simulink model "CrazyFlie_PosCntrl"  (R2015a)
settings: Solver=FixedStepDiscrete  SolverMode=SingleTasking  StartTime=0.0  StopTime=inf  FixedStep=0.02  RelTol=1e-3
PreLoadFcn:
  | addpath([cd filesep 'QuadCom']);
InitFcn:
  | %cd('..\Uart_Com');
libraries: simulink x2, CrazyFlie_lib x2
settings Model: CovSFcnEnable=off  Creator=Michael  LastModifiedBy=rshum
settings DataIOCC: SignalLoggingSaveFormat=ModelDataLogs
settings OptimizationCC: ExpressionDepthLimit=2147483647
settings DebuggingCC: UnderspecifiedInitializationDetection=Classic  MergeDetectMultiDrivingBlocksExec=none  SolverPrmCheckMsg=warning  FcnCallInpInsideContextMsg=UseLocalSettings  StateNameClashWarn=warning
settings HardwareCC: ProdLargestAtomicInteger=Long  ProdLargestAtomicFloat=Float  ProdHWDeviceType=ARM Compatible->ARM 7
settings SFSimCC: SimParseCustomCode=off
settings GRTTargetCC: CombineOutputUpdateFcns=off  GRTInterface=on

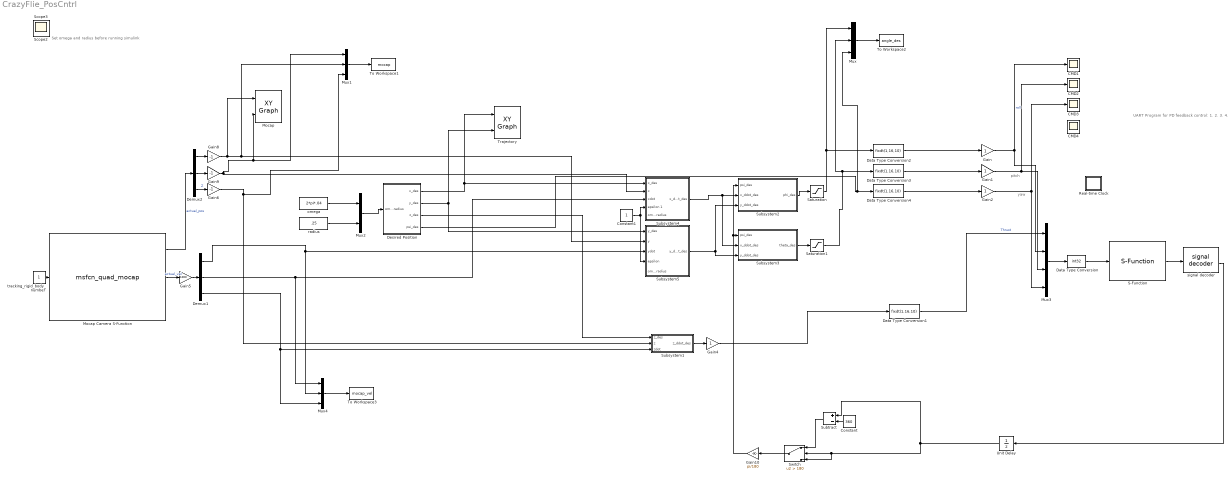
== system CrazyFlie_PosCntrl ==
  note: yaw
  note: pitch
  note: Set omega and radius before running simulink
  note: UART Program for PD feedback control:
      | 1.
      | 2.
      | 3.
      | 4.
  CMD{1..4} (4 alike) : Scope
      CMD1 settings: YMin=-1  YMax=1  SaveName=ScopeData15
      CMD2 settings: YMin=-0.15  YMax=0.15  SaveName=ScopeData16
      CMD3 settings: YMin=11.875  YMax=11.875  SaveName=ScopeData17
      CMD4 settings: YMin=11.875  YMax=11.875  SaveName=ScopeData18
  Constant : Constant  Value=360
  Constant1 : Constant
  Data Type Conversion : DataTypeConversion  OutDataTypeStr=int32  ConvertRealWorld=Stored Integer (SI)  SaturateOnIntegerOverflow=on
  Data Type Conversion{1..4} (4 alike) : DataTypeConversion  OutDataTypeStr=fixdt(1,16,10)
  Demux1 : Demux  Outputs=3
  Demux2 : Demux  Outputs=3
  "Desired Position " : Subsystem
  Gain : Gain  OutDataTypeStr=fixdt(1,16,10)
  Gain1 : Gain  OutDataTypeStr=fixdt(1,16,10)
  Gain10 : Gain  Gain=pi/180
  Gain2 : Gain  OutDataTypeStr=fixdt(1,16,10)
  Gain4 : Gain
  Gain5 : Gain  Gain=1000
  Gain6 : Gain  Gain=-1
  Gain8 : Gain  Gain=-1
  Gain9 : Gain  Gain=-1
  Mocap : simulink/Sinks/XY Graph  xmin=-1  xmax=1  ymin=-1  ymax=1  st=-1
  Mocap Camera S-Function : M-S-Function  FunctionName=msfcn_quad_mocap  mask(Mocap-Motion-Track){}
      mask Display:
      | image(imread('camera.png'))
      | color('white')
      | port_label('output', 1, 'Quad_Pos')
      | port_label('output', 2, 'Quad_Vel')
      | port_label('output', 3, 'Rel_Yaw')
      | port_label('input', 1, 'trackingBody_Num')
  Mux : Mux  Inputs=3
  Mux1 : Mux  Inputs=3
  Mux2 : Mux  Inputs=2
  Mux3 : Mux
  Mux4 : Mux  Inputs=3
  Real-time Clock : Subsystem  mask(Real-time Clock){sample_time=0.02, tolerance=1}
      mask prompts: sample_time "Synchronize with real-time every n seconds:"; tolerance "Real-time warning tolerance (seconds):"
      mask help: Real-time Synchronization Block
      mask Help: This block synchronizes simulation time with the PC real-time clock or UNIX system clock. The first dialog entry is the period at which the clock is checked to insure real-time synchronization. The second dialog entry is the number of seconds that the simulation time must be within real-time before a warning is printed.
      mask Display: plot(0,0,100,100,[40,60,60,54,54,64,69,76,82,77,81,83,83,81,78,74,70,64,57,49,41,35,32,30,30,31,34,40,47,47,40,40],[90,90,85,85,80,79,76,87,80,70,64,57,49,41,33,28,24,22,21,23,25,31,37,46,56,65,73,78,80,85,85,90],[69,53,53],[64,50,73])
  S-Function : CrazyFlie_lib/S-Function
  Saturation : Saturate  UpperLimit=1  LowerLimit=-1
  Saturation1 : Saturate  UpperLimit=1  LowerLimit=-1
  Subsystem1 : Subsystem
  Subsystem2 : Subsystem
  Subsystem3 : Subsystem
  Subsystem4 : Subsystem
  Subsystem5 : Subsystem
  Subtract : Sum  Inputs=+-
  Switch : Switch  Criteria=u2 > Threshold  Threshold=180
  To Workspace1 : ToWorkspace  VariableName=mocap  SaveFormat=Timeseries  SampleTime=-1
  To Workspace2 : ToWorkspace  VariableName=angle_des  SaveFormat=Timeseries  SampleTime=-1
  To Workspace3 : ToWorkspace  VariableName=mocap_vel  SaveFormat=Timeseries  SampleTime=-1
  "Trajectory " : simulink/Sinks/XY Graph  xmin=-1  xmax=1  ymin=-1  ymax=1  st=-1
  Unit Delay : UnitDelay  SampleTime=-1
  omega : Constant  Value=2*pi*.04
  radius : Constant  Value=.25
  signal decoder : CrazyFlie_lib/signal decoder
  tracking_rigid_body_number : Constant
  Scope2 : Scope
      settings: YMin=-0.09  YMax=0.07  SaveName=ScopeData2  MaxDataPoints=7500
  Scope3 : Scope
      settings: YMin=-1.25  YMax=2.75  SaveName=ScopeData3  MaxDataPoints=7500
  wires:
  Data Type Conversion/1 -> S-Function/1
  Mux3/1 -> Data Type Conversion/1
  Data Type Conversion2/1 -> Gain/1
  Data Type Conversion3/1 -> Gain1/1
  Data Type Conversion4/1 -> Gain2/1
  Gain/1 -> Mux3/2, CMD1/1  "roll"
  Gain1/1 -> Mux3/3, CMD2/1
  Gain2/1 -> Mux3/4, CMD3/1
  "Desired Position "/3(z_des) -> Subsystem1/1(z_des)
  Demux2/3 -> Gain6/1  "Z"
  Subsystem4/1(x_ddot_des) -> Subsystem3/2(x_ddot_des), Subsystem2/2(x_ddot_des)
  Subsystem5/1(y_ddot_des) -> Subsystem2/3("y_ddot_des "), Subsystem3/3("y_ddot_des ")
  "Desired Position "/2(y_des) -> "Trajectory "/2, Subsystem5/1(y_des)
  "Desired Position "/1(x_des) -> "Trajectory "/1, Subsystem4/1(x_des)
  Demux2/1 -> Gain8/1
  Demux2/2 -> Gain9/1
  tracking_rigid_body_number/1 -> Mocap Camera S-Function/1
  Mocap Camera S-Function/1 -> Demux2/1  "actual_pos"
  Mocap Camera S-Function/2 -> Gain5/1  "actual_vel"
  Subsystem3/1("theta_des ") -> Saturation1/1
  Subsystem2/1("phi_des ") -> Saturation/1
  Gain8/1 -> Mocap/1, Mux1/2, Subsystem5/2(y)
  Gain9/1 -> Mocap/2, Mux1/1, Subsystem4/2(x)
  Mux1/1 -> To Workspace1/1
  Demux1/1 -> Mux4/2, Subsystem5/3("ydot ")
  Demux1/2 -> Mux4/1, Subsystem4/3("xdot ")
  Gain5/1 -> Demux1/1
  Gain6/1 -> Subsystem1/2(z), Mux1/3
  Subsystem1/1(z_ddot_des) -> Gain4/1
  Mux4/1 -> To Workspace3/1
  signal decoder/3 -> Unit Delay/1
  Constant/1 -> Subtract/2
  Subtract/1 -> Switch/1
  Switch/1 -> Gain10/1
  Gain10/1 -> Subsystem3/1("psi_des "), Subsystem2/1("psi_des ")
  Unit Delay/1 -> Switch/3, Switch/2, Subtract/1
  Constant1/1 -> Subsystem4/4(epsilon 1), Subsystem5/4("epsilon ")
  Mux/1 -> To Workspace2/1
  "Desired Position "/4(psi_des) -> Mux/3, Data Type Conversion4/1
  Saturation1/1 -> Data Type Conversion3/1, Mux/2
  Saturation/1 -> Data Type Conversion2/1, Mux/1
  Demux1/3 -> Mux4/3, Subsystem1/3("zdot ")
  Data Type Conversion1/1 -> Mux3/1  "Thrust"
  Gain4/1 -> Data Type Conversion1/1
  Mux2/1 -> "Desired Position "/1("omg_radius ")
  omega/1 -> Mux2/1
  radius/1 -> Mux2/2
  S-Function/1 -> signal decoder/1

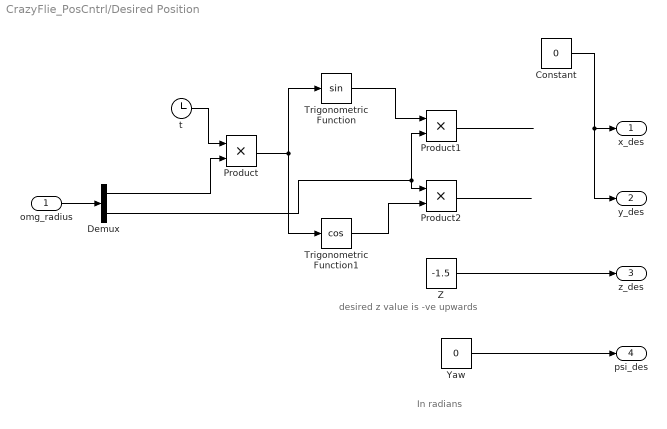
== system CrazyFlie_PosCntrl/Desired Position  ==
  note: desired z value
      | is -ve upwards
  note: In radians
  "omg_radius " : Inport
  Constant : Constant  Value=0
  Demux : Demux  Outputs=2
  Product : Product
  Product1 : Product
  Product2 : Product
  Trigonometric Function : Trigonometry
  Trigonometric Function1 : Trigonometry  Operator=cos
  Yaw : Constant  Value=0
  "Z " : Constant  Value=-1.5
  t : Clock
  x_des : Outport
  y_des : Outport  Port=2
  z_des : Outport  Port=3
  psi_des : Outport  Port=4
  wires:
  Yaw/1 -> psi_des/1
  "Z "/1 -> z_des/1
  Product2/1 -> ?
  Product1/1 -> ?
  t/1 -> Product/1
  Demux/1 -> Product/2
  Product/1 -> Trigonometric Function1/1, Trigonometric Function/1
  Demux/2 -> Product1/2, Product2/1
  Trigonometric Function/1 -> Product1/1
  Trigonometric Function1/1 -> Product2/2
  "omg_radius "/1 -> Demux/1
  Constant/1 -> y_des/1, x_des/1

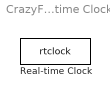
== system CrazyFlie_PosCntrl/Real-time Clock ==
  Real-time Clock : S-Function  FunctionName=rtclock  Parameters=sample_time, tolerance

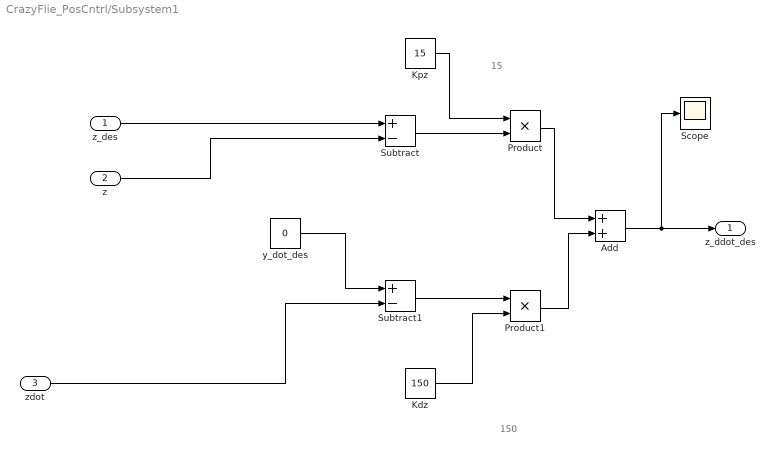
== system CrazyFlie_PosCntrl/Subsystem1 ==
  note: 15
  note: 150
  z_des : Inport
  z : Inport  Port=2
  "zdot " : Inport  Port=3
  Add : Sum
  "Kdz " : Constant  Value=150
  "Kpz " : Constant  Value=15
  Product : Product
  Product1 : Product
  Scope : Scope
      settings: YMin=-3  YMax=3  SaveName=ScopeData31
  Subtract : Sum  Inputs=+-
  Subtract1 : Sum  Inputs=+-
  y_dot_des : Constant  Value=0
  z_ddot_des : Outport
  wires:
  z/1 -> Subtract/2
  z_des/1 -> Subtract/1
  "Kpz "/1 -> Product/1
  Subtract/1 -> Product/2
  y_dot_des/1 -> Subtract1/1
  Subtract1/1 -> Product1/1
  "Kdz "/1 -> Product1/2
  Product1/1 -> Add/2
  Product/1 -> Add/1
  Add/1 -> Scope/1, z_ddot_des/1
  "zdot "/1 -> Subtract1/2

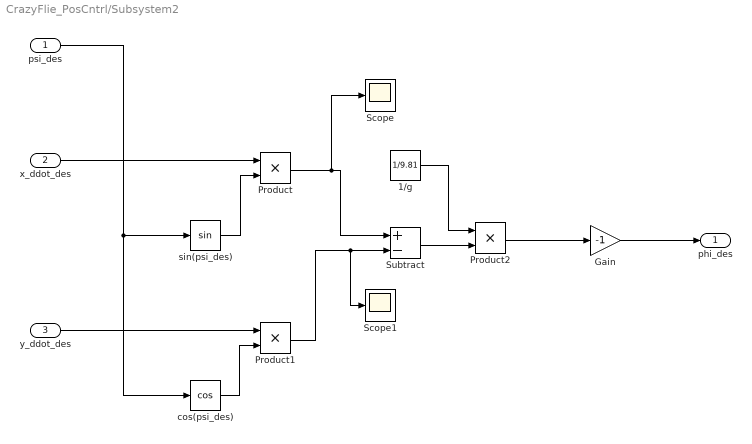
== system CrazyFlie_PosCntrl/Subsystem2 ==
  "psi_des " : Inport
  x_ddot_des : Inport  Port=2
  "y_ddot_des " : Inport  Port=3
  "1/g " : Constant  Value=1/9.81
  Gain : Gain  Gain=-1
  Product : Product
  Product1 : Product
  Product2 : Product
  Scope : Scope
      settings: TimeRange=30  YMin=-30  YMax=20  SaveName=ScopeData28
  Scope1 : Scope
      settings: TimeRange=30  YMin=-61.5  YMax=-61.3  SaveName=ScopeData30
  Subtract : Sum  Inputs=+-
  cos(psi_des) : Trigonometry  Operator=cos
  sin(psi_des) : Trigonometry
  "phi_des " : Outport
  wires:
  "psi_des "/1 -> sin(psi_des)/1, cos(psi_des)/1
  x_ddot_des/1 -> Product/1
  sin(psi_des)/1 -> Product/2
  cos(psi_des)/1 -> Product1/2
  "y_ddot_des "/1 -> Product1/1
  Product/1 -> Scope/1, Subtract/1
  Product1/1 -> Scope1/1, Subtract/2
  Subtract/1 -> Product2/2
  "1/g "/1 -> Product2/1
  Product2/1 -> Gain/1
  Gain/1 -> "phi_des "/1

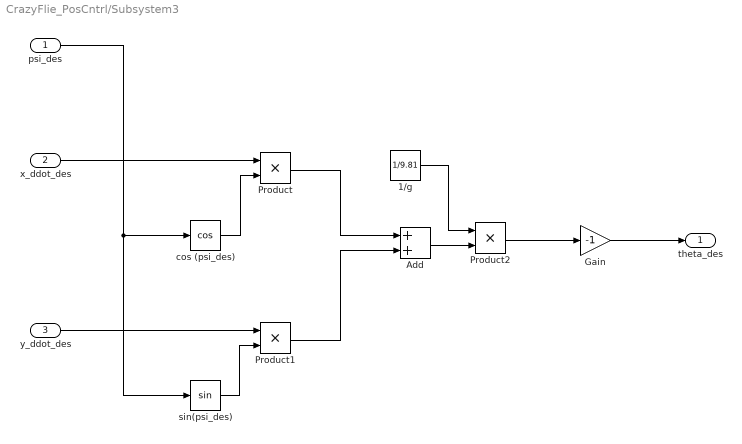
== system CrazyFlie_PosCntrl/Subsystem3 ==
  "psi_des " : Inport
  x_ddot_des : Inport  Port=2
  "y_ddot_des " : Inport  Port=3
  "1/g " : Constant  Value=1/9.81
  Add : Sum
  Gain : Gain  Gain=-1
  Product : Product
  Product1 : Product
  Product2 : Product
  cos (psi_des) : Trigonometry  Operator=cos
  sin(psi_des) : Trigonometry
  "theta_des " : Outport
  wires:
  "psi_des "/1 -> cos (psi_des)/1, sin(psi_des)/1
  x_ddot_des/1 -> Product/1
  cos (psi_des)/1 -> Product/2
  sin(psi_des)/1 -> Product1/2
  "y_ddot_des "/1 -> Product1/1
  Product/1 -> Add/1
  Product1/1 -> Add/2
  Add/1 -> Product2/2
  "1/g "/1 -> Product2/1
  Product2/1 -> Gain/1
  Gain/1 -> "theta_des "/1

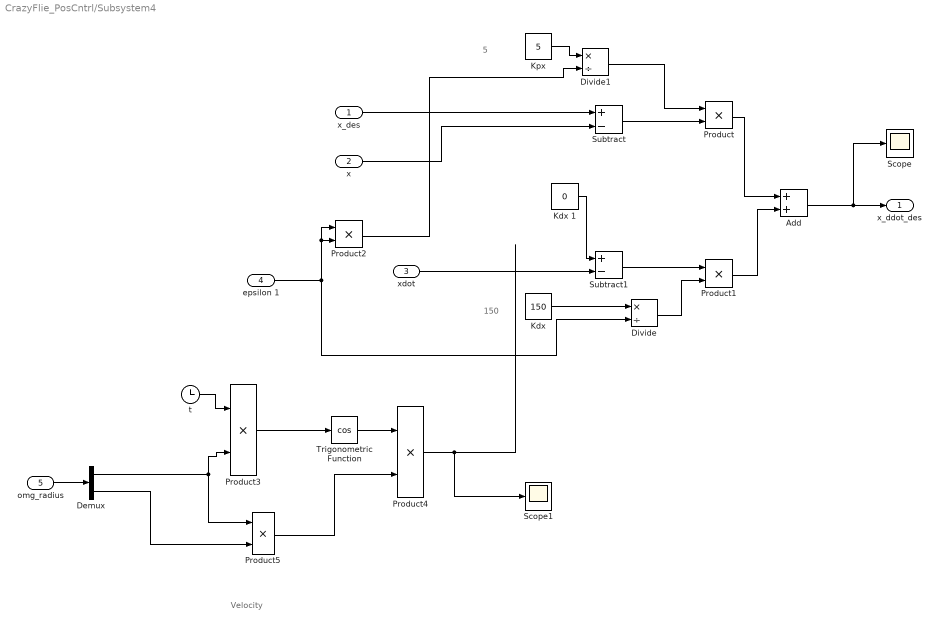
== system CrazyFlie_PosCntrl/Subsystem4 ==
  note: Velocity
  note: 150
  note: 5
  x_des : Inport
  x : Inport  Port=2
  "xdot " : Inport  Port=3
  epsilon 1 : Inport  Port=4
  "omg_radius " : Inport  Port=5
  Add : Sum
  Demux : Demux  Outputs=2
  Divide : Product  Inputs=*/
  Divide1 : Product  Inputs=*/
  "Kdx " : Constant  Value=150
  Kdx 1 : Constant  Value=0
  Kpx : Constant  Value=5
  Product{,1..5} (6 alike) : Product
  Scope : Scope
      settings: TimeRange=50  YMin=-4.5  YMax=-1.5  SaveName=ScopeData29
  Scope1 : Scope
      settings: TimeRange=45  YMin=-0.1  YMax=0.1  SaveName=ScopeData33
  Subtract : Sum  Inputs=+-
  Subtract1 : Sum  Inputs=+-
  Trigonometric Function : Trigonometry  Operator=cos
  "t " : Clock
  x_ddot_des : Outport
  wires:
  x/1 -> Subtract/2
  "xdot "/1 -> Subtract1/2
  x_des/1 -> Subtract/1
  Subtract/1 -> Product/2
  Subtract1/1 -> Product1/1
  Product1/1 -> Add/2
  Product/1 -> Add/1
  Add/1 -> Scope/1, x_ddot_des/1
  epsilon 1/1 -> Product2/1, Product2/2, Divide/2
  Product2/1 -> Divide1/2
  Kpx/1 -> Divide1/1
  "Kdx "/1 -> Divide/1
  Divide/1 -> Product1/2
  Divide1/1 -> Product/1
  "t "/1 -> Product3/1
  Product3/1 -> Trigonometric Function/1
  Trigonometric Function/1 -> Product4/1
  Demux/1 -> Product3/2, Product5/1
  Demux/2 -> Product5/2
  Product5/1 -> Product4/2
  "omg_radius "/1 -> Demux/1
  Product4/1 -> Scope1/1
  Kdx 1/1 -> Subtract1/1

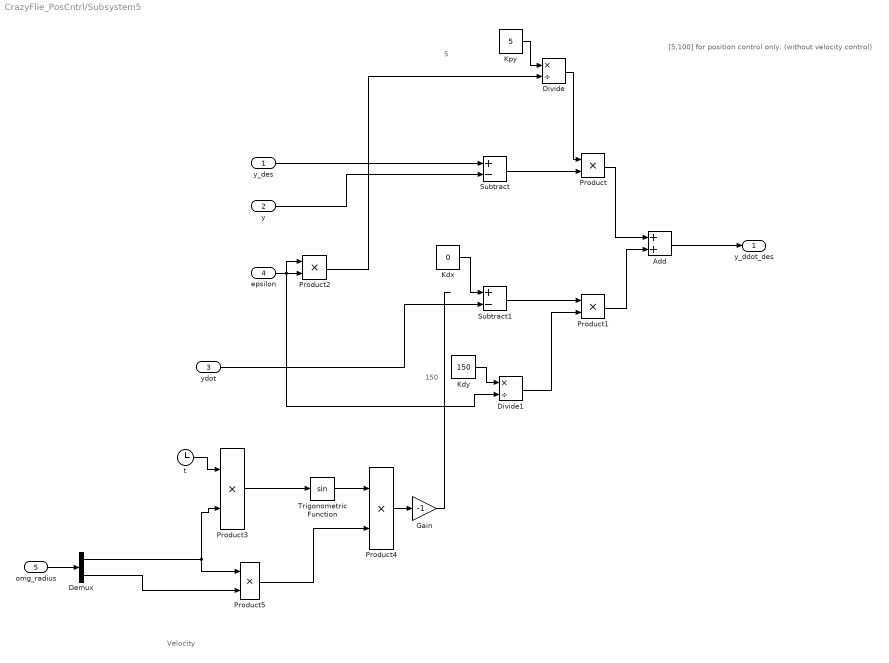
== system CrazyFlie_PosCntrl/Subsystem5 ==
  note: Velocity
  note: [5,100] for position control only. (without velocity control)
  note: 150
  note: 5
  y_des : Inport
  y : Inport  Port=2
  "ydot " : Inport  Port=3
  "epsilon " : Inport  Port=4
  "omg_radius " : Inport  Port=5
  Add : Sum
  Demux : Demux  Outputs=2
  Divide : Product  Inputs=*/
  Divide1 : Product  Inputs=*/
  Gain : Gain  Gain=-1
  "Kdx " : Constant  Value=0
  "Kdy " : Constant  Value=150
  Kpy : Constant  Value=5
  Product{,1..5} (6 alike) : Product
  Subtract : Sum  Inputs=+-
  Subtract1 : Sum  Inputs=+-
  Trigonometric Function : Trigonometry
  "t " : Clock
  y_ddot_des : Outport
  wires:
  y/1 -> Subtract/2
  y_des/1 -> Subtract/1
  Subtract/1 -> Product/2
  Product4/1 -> Gain/1
  Subtract1/1 -> Product1/1
  Product1/1 -> Add/2
  Product/1 -> Add/1
  Add/1 -> y_ddot_des/1
  "ydot "/1 -> Subtract1/2
  Divide/1 -> Product/1
  Kpy/1 -> Divide/1
  "Kdy "/1 -> Divide1/1
  Divide1/1 -> Product1/2
  "epsilon "/1 -> Divide1/2, Product2/1, Product2/2
  Product2/1 -> Divide/2
  "t "/1 -> Product3/1
  Product3/1 -> Trigonometric Function/1
  Trigonometric Function/1 -> Product4/1
  Gain/1 -> ?
  Demux/1 -> Product3/2, Product5/1
  Demux/2 -> Product5/2
  Product5/1 -> Product4/2
  "omg_radius "/1 -> Demux/1
  "Kdx "/1 -> Subtract1/1
